simulink library "libLgBattery"  (R2020a)
settings: Solver=VariableStepAuto  StartTime=0.0  StopTime=10.0  RelTol=1e-3
undefined symbols (not defined in the file): Ion, Lithium
libraries: powerlib x2, $bdroot x1, electricdrivelib x1
settings Model: Creator=pkoralew  LastModifiedBy=pkoralew

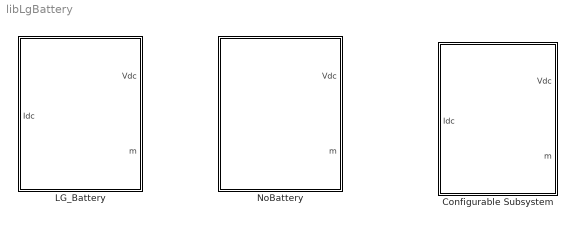
== system libLgBattery ==
  Configurable Subsystem : Subsystem  BlockChoice=LG_Battery
      settings: TemplateBlock=self  MemberBlocks=LG_Battery,NoBattery
  LG_Battery : Subsystem
  NoBattery : Subsystem

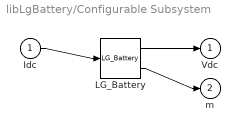
== system libLgBattery/Configurable Subsystem ==
  Idc : Inport
  LG_Battery : $bdroot/LG_Battery  SystemSampleTime=-1  Latency=0  AutoFrameSizeCalculation=off
  Vdc : Outport
  m : Outport  Port=2
  wires:
  Idc/1 -> LG_Battery/1
  LG_Battery/1 -> Vdc/1
  LG_Battery/2 -> m/1

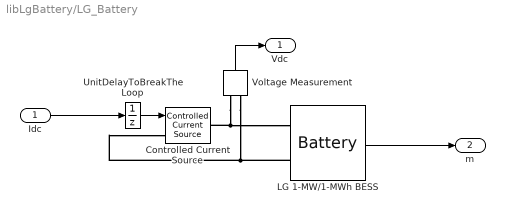
== system libLgBattery/LG_Battery ==
  Idc : Inport
  Controlled Current Source : powerlib/Electrical Sources/Controlled Current Source  Initialize=on  Source_Type=AC  Amplitude=0  Phase=0  Frequency=0  Measurements=None
  LG 1-MW/1-MWh BESS : electricdrivelib/Extra Sources/Battery  BatType=Lithium-Ion  ShowTempParam=off  ThermalPreset=no  ShowAgeParam=off  NomV=1000  NomQ=1e3  SOC=80  Batt_Tr=0.001  PresetModel=on  MaxQ=1000  MinV=750  FullV=1163.9871  Dis_rate=434.7826  R=0.01  Normal_OP=904.3478  expZone="[1080.3859      49.130435]"  current=[250 500 1000]  Units=Time  Tci=20  NomT=20  T2=-30  MaxQ2=4.8  FullV2=7.1  Normal_OP2=5.655  expZone2="[6.58           1]"  Rca=0.6  ti=2000  Dp=0  Neq0=0  Tsim=1e6  Ta1=25  Qeol=5.4*0.9  Reol=0.013333*1.2  Char_age=[2.3478, 3]  Dis_age=[2.3478, 10]  N1=1500  N2=10500  N3=1000  N4=1400  Ta2=45  N5=950
  UnitDelayToBreakTheLoop : UnitDelay  InitialCondition=1000  SampleTime=-1  HasFrameUpgradeWarning=on
  Voltage Measurement : powerlib/Measurements/Voltage Measurement  PhasorSimulation=off  OutputType=Complex  PSBequivalent=0
  Vdc : Outport
  m : Outport  Port=2
  wires:
  Idc/1 -> UnitDelayToBreakTheLoop/1
  LG 1-MW/1-MWh BESS/1 -> m/1
  UnitDelayToBreakTheLoop/1 -> Controlled Current Source/1
  Voltage Measurement/1 -> Vdc/1
  connections:
  Voltage Measurement/LConn1 -- Controlled Current Source/RConn1 -- LG 1-MW/1-MWh BESS/LConn1
  Voltage Measurement/LConn2 -- LG 1-MW/1-MWh BESS/LConn2 -- Controlled Current Source/LConn1

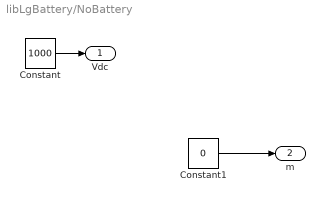
== system libLgBattery/NoBattery ==
  Constant : Constant  Value=1000
  Constant1 : Constant  Value=0
  Vdc : Outport
  m : Outport  Port=2
  wires:
  Constant1/1 -> m/1
  Constant/1 -> Vdc/1
